simulink model "fullstatefeedback"  (R2023a)
settings: Solver=VariableStepAuto  StartTime=0.0  StopTime=10.0  RelTol=1e-3
undefined symbols (not defined in the file): A, B, C, C_o, g, I_noload, init, J_observer, K_cont_int, K_cont_x, K_disc_int, K_disc_x, K_m, l, m, min_sampling_time, R, sys_disc, x1_bar, x2_bar
settings Model: Creator=yunzh  LastModifiedBy=yunzh

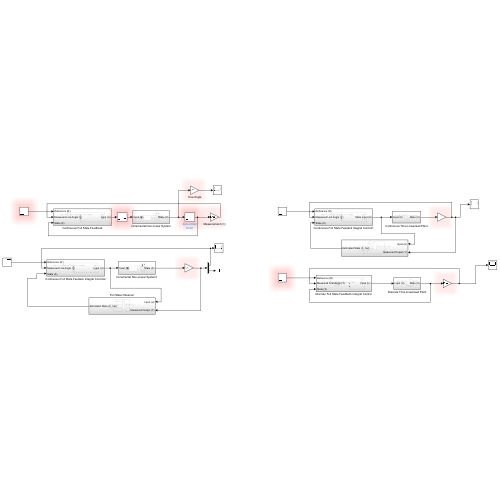
[thumbnail: Simulink's stored preview of the top-level diagram]
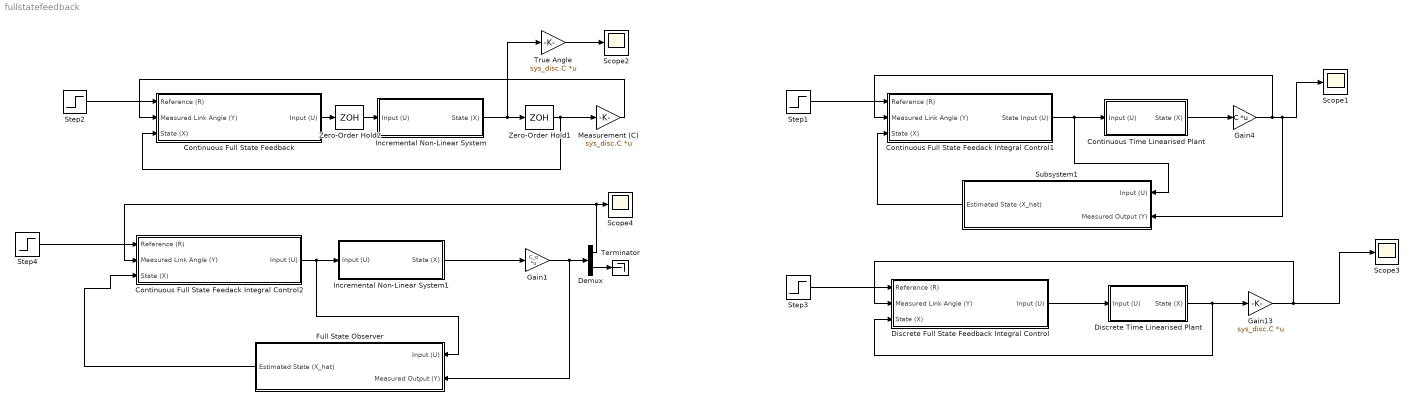
== system fullstatefeedback ==
  Continuous Full State Feedack Integral Control1 : Subsystem
  Continuous Full State Feedack Integral Control2 : Subsystem
  Continuous Full State Feedback : Subsystem
  Continuous Time Linearised Plant : Subsystem
  Demux : Demux  Outputs=2
  Discrete Full State Feedback Integral Control : Subsystem
  Discrete Time Linearised Plant : Subsystem
  Full State Observer : Subsystem
  Gain1 : Gain  Gain=C_o  Multiplication=Matrix(K*u)
  Gain13 : Gain  Gain=sys_disc.C  Multiplication=Matrix(K*u)
  Gain4 : Gain  Gain=C  Multiplication=Matrix(K*u)
  Incremental Non-Linear System : Subsystem
  Incremental Non-Linear System1 : Subsystem
  Measurement (C) : Gain  Gain=sys_disc.C  Multiplication=Matrix(K*u)
  Scope{1..4} (4 alike) : Scope
  Step1 : Step  Time=0  After=0.5  SampleTime=0
  Step2 : Step  Time=0  After=0.5  SampleTime=min_sampling_time
  Step3 : Step  Time=0  After=0.5  SampleTime=min_sampling_time
  Step4 : Step  Time=0  After=deg2rad(15)  SampleTime=0
  Subsystem1 : Subsystem
  Terminator : Terminator
  True Angle : Gain  Gain=sys_disc.C  Multiplication=Matrix(K*u)
  Zero-Order Hold1 : ZeroOrderHold  SampleTime=min_sampling_time
  Zero-Order Hold2 : ZeroOrderHold  SampleTime=min_sampling_time
  wires:
  Gain4/1 -> Continuous Full State Feedack Integral Control1/2(Measured Link Angle (Y)), Subsystem1/2(Measured Output (Y)), Scope1/1
  Gain13/1 -> Discrete Full State Feedback Integral Control/2(Measured Link Angle (Y)), Scope3/1
  Continuous Time Linearised Plant/1(State (X)) -> Gain4/1
  Step1/1 -> Continuous Full State Feedack Integral Control1/1(Reference (R))
  Continuous Full State Feedack Integral Control1/1(State Input (U)) -> Subsystem1/1(Input (U)), Continuous Time Linearised Plant/1(Input (U))
  Discrete Time Linearised Plant/1(State (X)) -> Gain13/1, Discrete Full State Feedback Integral Control/3(State (X))
  Step3/1 -> Discrete Full State Feedback Integral Control/1(Reference (R))
  Discrete Full State Feedback Integral Control/1(Input (U)) -> Discrete Time Linearised Plant/1(Input (U))
  Continuous Full State Feedack Integral Control2/1(Input (U)) -> Full State Observer/1(Input (U)), Incremental Non-Linear System1/1(Input (U))
  Incremental Non-Linear System1/1(State (X)) -> Gain1/1
  Gain1/1 -> Full State Observer/2(Measured Output (Y)), Demux/1
  Full State Observer/1(Estimated State (X_hat)) -> Continuous Full State Feedack Integral Control2/3(State (X))
  Step4/1 -> Continuous Full State Feedack Integral Control2/1(Reference (R))
  Subsystem1/1(Estimated State (X_hat)) -> Continuous Full State Feedack Integral Control1/3(State (X))
  Zero-Order Hold2/1 -> Incremental Non-Linear System/1(Input (U))
  Step2/1 -> Continuous Full State Feedback/1(Reference (R))
  Continuous Full State Feedback/1(Input (U)) -> Zero-Order Hold2/1
  Zero-Order Hold1/1 -> Continuous Full State Feedback/3(State (X)), Measurement (C)/1
  Measurement (C)/1 -> Continuous Full State Feedback/2(Measured Link Angle (Y))
  Incremental Non-Linear System/1(State (X)) -> True Angle/1, Zero-Order Hold1/1
  Demux/1 -> Scope4/1, Continuous Full State Feedack Integral Control2/2(Measured Link Angle (Y))
  Demux/2 -> Terminator/1
  True Angle/1 -> Scope2/1

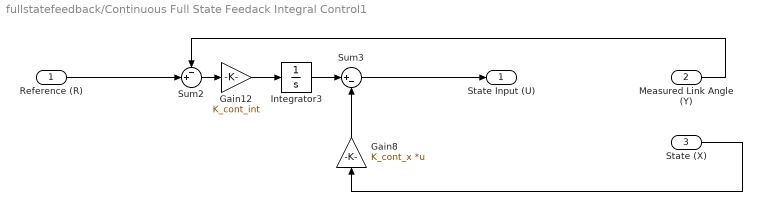
== system fullstatefeedback/Continuous Full State Feedack Integral Control1 ==
  Reference (R) : Inport
  Measured Link Angle (Y) : Inport  Port=2
  State (X) : Inport  Port=3
  Gain12 : Gain  Gain=K_cont_int
  Gain8 : Gain  Gain=K_cont_x  Multiplication=Matrix(K*u)
  Integrator3 : Integrator
  Sum2 : Sum  Inputs=-+|
  Sum3 : Sum  Inputs=|+-
  State Input (U) : Outport
  wires:
  Sum2/1 -> Gain12/1
  Gain8/1 -> Sum3/2
  Integrator3/1 -> Sum3/1
  Gain12/1 -> Integrator3/1
  Reference (R)/1 -> Sum2/2
  Sum3/1 -> State Input (U)/1
  Measured Link Angle (Y)/1 -> Sum2/1
  State (X)/1 -> Gain8/1

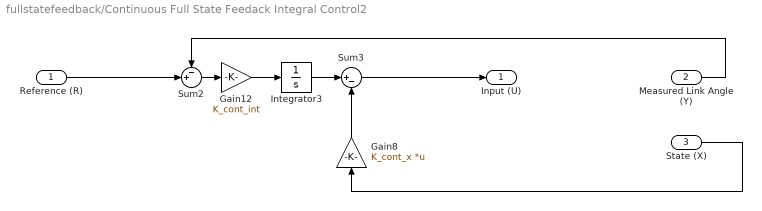
== system fullstatefeedback/Continuous Full State Feedack Integral Control2 ==
  Reference (R) : Inport
  Measured Link Angle (Y) : Inport  Port=2
  State (X) : Inport  Port=3
  Gain12 : Gain  Gain=K_cont_int
  Gain8 : Gain  Gain=K_cont_x  Multiplication=Matrix(K*u)
  Integrator3 : Integrator
  Sum2 : Sum  Inputs=-+|
  Sum3 : Sum  Inputs=|+-
  Input (U) : Outport
  wires:
  Sum2/1 -> Gain12/1
  Gain8/1 -> Sum3/2
  Integrator3/1 -> Sum3/1
  Gain12/1 -> Integrator3/1
  Reference (R)/1 -> Sum2/2
  Sum3/1 -> Input (U)/1
  Measured Link Angle (Y)/1 -> Sum2/1
  State (X)/1 -> Gain8/1

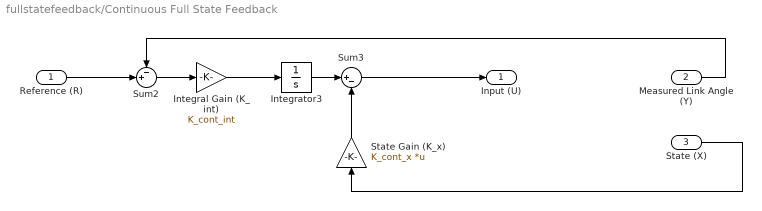
== system fullstatefeedback/Continuous Full State Feedback ==
  Reference (R) : Inport
  Measured Link Angle (Y) : Inport  Port=2
  State (X) : Inport  Port=3
  Integral Gain (K_int) : Gain  Gain=K_cont_int
  Integrator3 : Integrator
  State Gain (K_x) : Gain  Gain=K_cont_x  Multiplication=Matrix(K*u)
  Sum2 : Sum  Inputs=-+|
  Sum3 : Sum  Inputs=|+-
  Input (U) : Outport
  wires:
  Sum2/1 -> Integral Gain (K_int)/1
  State Gain (K_x)/1 -> Sum3/2
  Integrator3/1 -> Sum3/1
  Integral Gain (K_int)/1 -> Integrator3/1
  Reference (R)/1 -> Sum2/2
  Sum3/1 -> Input (U)/1
  Measured Link Angle (Y)/1 -> Sum2/1
  State (X)/1 -> State Gain (K_x)/1

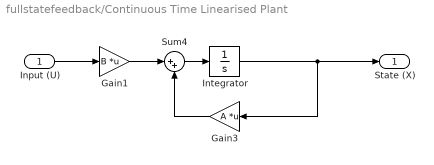
== system fullstatefeedback/Continuous Time Linearised Plant ==
  Input (U) : Inport
  Gain1 : Gain  Gain=B  Multiplication=Matrix(K*u)
  Gain3 : Gain  Gain=A  Multiplication=Matrix(K*u)
  Integrator : Integrator
  Sum4 : Sum  Inputs=|++
  State (X) : Outport
  wires:
  Input (U)/1 -> Gain1/1
  Integrator/1 -> State (X)/1, Gain3/1
  Gain3/1 -> Sum4/2
  Gain1/1 -> Sum4/1
  Sum4/1 -> Integrator/1

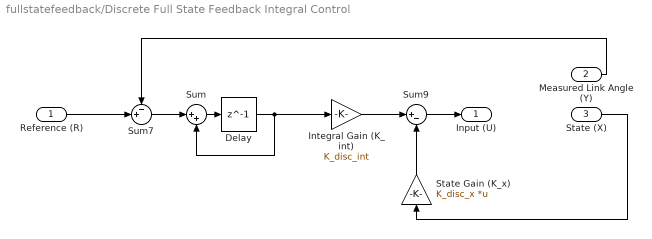
== system fullstatefeedback/Discrete Full State Feedback Integral Control ==
  Reference (R) : Inport
  Measured Link Angle (Y) : Inport  Port=2
  State (X) : Inport  Port=3
  Delay : Delay  DelayLength=1  SampleTime=min_sampling_time
  Integral Gain (K_int) : Gain  Gain=K_disc_int
  State Gain (K_x) : Gain  Gain=K_disc_x  Multiplication=Matrix(K*u)
  Sum : Sum  Inputs=|++
  Sum7 : Sum  Inputs=-+|
  Sum9 : Sum  Inputs=|+-
  Input (U) : Outport
  wires:
  Integral Gain (K_int)/1 -> Sum9/1
  Reference (R)/1 -> Sum7/2
  Sum/1 -> Delay/1
  State Gain (K_x)/1 -> Sum9/2
  Sum7/1 -> Sum/1
  Delay/1 -> Sum/2, Integral Gain (K_int)/1
  Sum9/1 -> Input (U)/1
  State (X)/1 -> State Gain (K_x)/1
  Measured Link Angle (Y)/1 -> Sum7/1

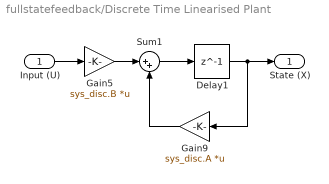
== system fullstatefeedback/Discrete Time Linearised Plant ==
  Input (U) : Inport
  Delay1 : Delay  DelayLength=1  SampleTime=min_sampling_time
  Gain5 : Gain  Gain=sys_disc.B  Multiplication=Matrix(K*u)
  Gain9 : Gain  Gain=sys_disc.A  Multiplication=Matrix(K*u)
  Sum1 : Sum  Inputs=|++
  State (X) : Outport
  wires:
  Gain9/1 -> Sum1/2
  Gain5/1 -> Sum1/1
  Sum1/1 -> Delay1/1
  Delay1/1 -> Gain9/1, State (X)/1
  Input (U)/1 -> Gain5/1

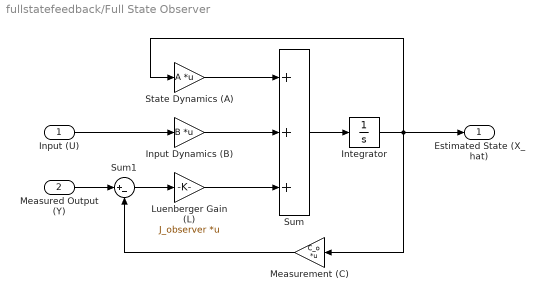
== system fullstatefeedback/Full State Observer ==
  Input (U) : Inport
  Measured Output (Y) : Inport  Port=2
  Input Dynamics (B) : Gain  Gain=B  Multiplication=Matrix(K*u)
  Integrator : Integrator
  Luenberger Gain (L) : Gain  Gain=J_observer  Multiplication=Matrix(K*u)
  Measurement (C) : Gain  Gain=C_o  Multiplication=Matrix(K*u)
  State Dynamics (A) : Gain  Gain=A  Multiplication=Matrix(K*u)
  Sum : Sum  Inputs=+++
  Sum1 : Sum  Inputs=|+-
  Estimated State (X_hat) : Outport
  wires:
  Input (U)/1 -> Input Dynamics (B)/1
  Measured Output (Y)/1 -> Sum1/1
  Input Dynamics (B)/1 -> Sum/2
  Sum/1 -> Integrator/1
  Measurement (C)/1 -> Sum1/2
  Sum1/1 -> Luenberger Gain (L)/1
  Luenberger Gain (L)/1 -> Sum/3
  State Dynamics (A)/1 -> Sum/1
  Integrator/1 -> Estimated State (X_hat)/1, State Dynamics (A)/1, Measurement (C)/1

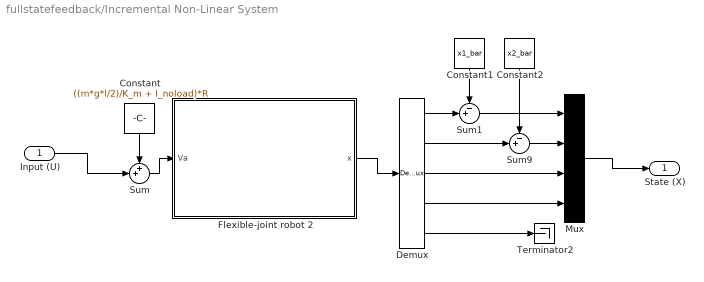
== system fullstatefeedback/Incremental Non-Linear System ==
  Input (U) : Inport
  Constant : Constant  Value=((m*g*l/2)/K_m + I_noload)*R
  Constant1 : Constant  Value=x1_bar
  Constant2 : Constant  Value=x2_bar
  Demux : Demux  Outputs=5
  Flexible-joint robot 2 : Subsystem
      mask Display: image('$imagefile'); % Use "Edit Image" on toolstrip to change.
  Mux : Mux
  Sum : Sum  Inputs=++|
  Sum1 : Sum  Inputs=-+|
  Sum9 : Sum  Inputs=-+|
  Terminator2 : Terminator
  State (X) : Outport
  wires:
  Flexible-joint robot 2/1(x) -> Demux/1
  Demux/1 -> Sum1/2
  Demux/2 -> Sum9/2
  Demux/5 -> Terminator2/1
  Sum/1 -> Flexible-joint robot 2/1(Va)
  Constant1/1 -> Sum1/1
  Sum9/1 -> Mux/2
  Constant2/1 -> Sum9/1
  Sum1/1 -> Mux/1
  Demux/4 -> Mux/4
  Demux/3 -> Mux/3
  Constant/1 -> Sum/1
  Input (U)/1 -> Sum/2
  Mux/1 -> State (X)/1

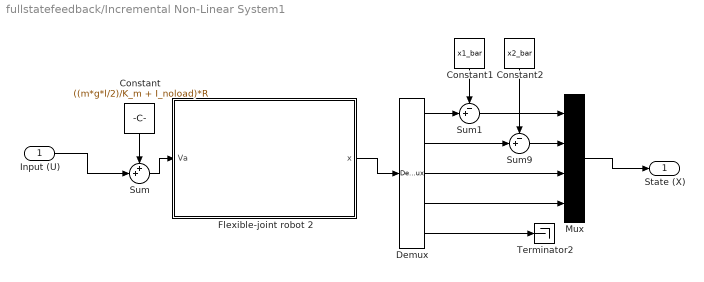
== system fullstatefeedback/Incremental Non-Linear System1 ==
  Input (U) : Inport
  Constant : Constant  Value=((m*g*l/2)/K_m + I_noload)*R
  Constant1 : Constant  Value=x1_bar
  Constant2 : Constant  Value=x2_bar
  Demux : Demux  Outputs=5
  Flexible-joint robot 2 : Subsystem
      mask Display: image('$imagefile'); % Use "Edit Image" on toolstrip to change.
  Mux : Mux
  Sum : Sum  Inputs=++|
  Sum1 : Sum  Inputs=-+|
  Sum9 : Sum  Inputs=-+|
  Terminator2 : Terminator
  State (X) : Outport
  wires:
  Flexible-joint robot 2/1(x) -> Demux/1
  Demux/1 -> Sum1/2
  Demux/2 -> Sum9/2
  Demux/5 -> Terminator2/1
  Sum/1 -> Flexible-joint robot 2/1(Va)
  Constant1/1 -> Sum1/1
  Sum9/1 -> Mux/2
  Constant2/1 -> Sum9/1
  Sum1/1 -> Mux/1
  Demux/4 -> Mux/4
  Demux/3 -> Mux/3
  Constant/1 -> Sum/1
  Input (U)/1 -> Sum/2
  Mux/1 -> State (X)/1

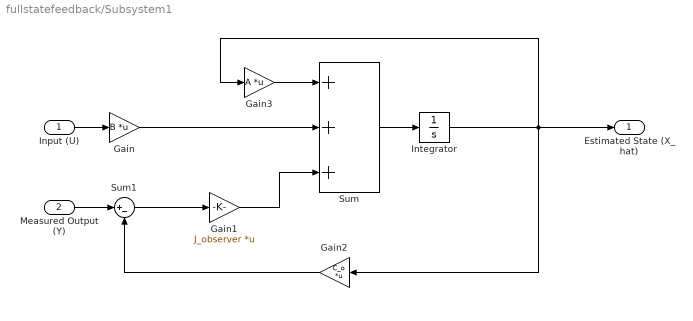
== system fullstatefeedback/Subsystem1 ==
  Input (U) : Inport
  Measured Output (Y) : Inport  Port=2
  Gain : Gain  Gain=B  Multiplication=Matrix(K*u)
  Gain1 : Gain  Gain=J_observer  Multiplication=Matrix(K*u)
  Gain2 : Gain  Gain=C_o  Multiplication=Matrix(K*u)
  Gain3 : Gain  Gain=A  Multiplication=Matrix(K*u)
  Integrator : Integrator
  Sum : Sum  Inputs=+++
  Sum1 : Sum  Inputs=|+-
  Estimated State (X_hat) : Outport
  wires:
  Input (U)/1 -> Gain/1
  Measured Output (Y)/1 -> Sum1/1
  Gain/1 -> Sum/2
  Sum/1 -> Integrator/1
  Gain2/1 -> Sum1/2
  Sum1/1 -> Gain1/1
  Gain1/1 -> Sum/3
  Gain3/1 -> Sum/1
  Integrator/1 -> Gain2/1, Gain3/1, Estimated State (X_hat)/1

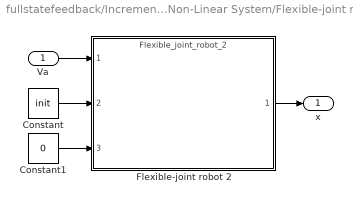
== system fullstatefeedback/Incremental Non-Linear System/Flexible-joint robot 2 ==
  Va : Inport
  Constant : Constant  Value=init
  Constant1 : Constant  Value=0
  Flexible-joint robot 2 : ModelReference  ModelNameDialog=Flexible_joint_robot_2  ModelReferenceVersion=1.65  CopyOfModelProtected=on
  x : Outport
  wires:
  Va/1 -> Flexible-joint robot 2/1
  Constant1/1 -> Flexible-joint robot 2/3
  Constant/1 -> Flexible-joint robot 2/2
  Flexible-joint robot 2/1 -> x/1

== system fullstatefeedback/Incremental Non-Linear System1/Flexible-joint robot 2 ==
  Va : Inport
  Constant : Constant  Value=init
  Constant1 : Constant  Value=0
  Flexible-joint robot 2 : ModelReference  ModelNameDialog=Flexible_joint_robot_2  ModelReferenceVersion=1.65  CopyOfModelProtected=on
  x : Outport
  wires:
  Va/1 -> Flexible-joint robot 2/1
  Constant1/1 -> Flexible-joint robot 2/3
  Constant/1 -> Flexible-joint robot 2/2
  Flexible-joint robot 2/1 -> x/1
